simulink model "Project_design_1"  (R2019a)
settings: Solver=FixedStepAuto  StartTime=0.0  StopTime=20.0  FixedStep=0.001  RelTol=1e-3
libraries: simulink_extras x1
settings Model: Creator=ChairmanYang1966  LastModifiedBy=ChairmanYang1966

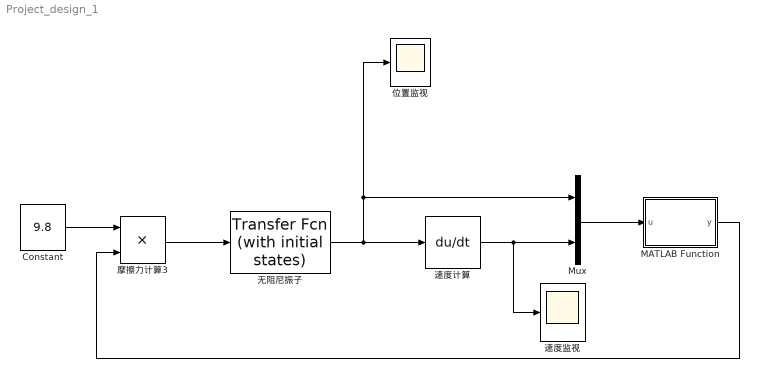
== system Project_design_1 ==
  Constant : Constant  Value=9.8
  MATLAB Function : MATLAB Function  TreatAsAtomicUnit=on
  Mux : Mux  Inputs=2
  位置监视 : Scope
  摩擦力计算3 : Product
  无阻尼振子 : simulink_extras/Additional Linear/Transfer Fcn (with initial states)  N=[1]  D="[10  0  1000]"  X0=[0 10]
  速度监视 : Scope
  速度计算 : Derivative
  wires:
  Constant/1 -> 摩擦力计算3/1
  无阻尼振子/1 -> 速度计算/1, 位置监视/1, Mux/1
  摩擦力计算3/1 -> 无阻尼振子/1
  Mux/1 -> MATLAB Function/1(u)
  速度计算/1 -> 速度监视/1, Mux/2
  MATLAB Function/1(y) -> 摩擦力计算3/2

== matlab function Project_design_1/MATLAB Function ==
  data: u input; y output
function y = fcn(u)
if u(2)~=0
    y=-u(2)/abs(u(2));
else
    if abs(1000*u(1))>9.8
        y=-u(1)/abs(u(1));
    else
        y=0;
    end
end
